simulink model "SICARO_STALL"  (R2022b)
settings: Solver=ode23t  StartTime=0.0  StopTime=84  MaxStep=1e-3  RelTol=1e-3  AbsTol=1e-3
values from neighbouring files (symbols this model uses):
  air_rho = 1.225    [sicaro_inherited_params(stall).mat]
  battery_capacity = 22.8    [sicaro_inherited_params(stall).mat]
  CDO = 10.25    [sicaro_inherited_params(stall).mat]
  drag_linear = 0.002    [sicaro_inherited_params(stall).mat]
  drag_quad = 0.005    [sicaro_inherited_params(stall).mat]
  filtD_motor = 100    [sicaro_inherited_params(stall).mat]
  filtSpd_motor = 0.001    [sicaro_inherited_params(stall).mat]
  flap_radius = 0.05312    [sicaro_inherited_params(stall).mat]
  flap_surface_area = 0.025    [sicaro_inherited_params(stall).mat]
  kd_motor = 0    [sicaro_inherited_params(stall).mat]
  ki_motor = 0.00045    [sicaro_inherited_params(stall).mat]
  klinear = 0.03    [sicaro_inherited_params(stall).mat]
  kquad = 0.025    [sicaro_inherited_params(stall).mat]
  limit_motor = 0.25    [sicaro_inherited_params(stall).mat]
  monoco_mass = 160    [sicaro_inherited_params(stall).mat]
  monoco_prop =     [sicaro_inherited_params(stall).mat]
  monoco_radius = 0.61    [sicaro_inherited_params(stall).mat]
  monoco_wing =     [sicaro_inherited_params(stall).mat]
  monoco_wing_area = 0.239    [sicaro_inherited_params(stall).mat]
  waypoints = [-2 -2 0.14 -2 -2 6 0 0 6 2 0 6 ... (15 elements, 3x5)]    [sicaro_inherited_params(stall).mat]
undefined symbols (not defined in the file or in its folder): X, Y, Z
libraries: sm_lib x96, nesl_utility x38, slpidlib x22, fl_lib x12, sdl_lib x3, simulink x2, simulink_extras x1, batteryecm_lib x1, ee_lib x1
(part 8 of 8)

== matlab function SICARO_STALL/Monowing/Monowing_Assem/Cyclic Command Distribution (Disk-Pitch Body-Roll) abt Yw ==
  data: azi input; quadrant input; flap_dihedral_pitch_cmd output; gain_disk_pitch input; Toggle input; Motor_Pulse output; desired_heading input
function [flap_dihedral_pitch_cmd,Motor_Pulse] = fcn(azi, quadrant, gain_disk_pitch, Toggle, desired_heading)

upper_bound = zeros(1,1);
lower_bound = zeros(1,1);
azimuth = azi;
heading = desired_heading;
pitch = zeros(1,1);
Motor_Pulse = zeros(1,1);
%% Quadrants anti clockwise fashion

if quadrant == 0 
    upper_bound = pi/2 + pi/4; 
    lower_bound = pi/2 - pi/4;
    if abs(azimuth) < upper_bound && abs(azimuth) > lower_bound
        tilt_xw = sin(azimuth); % tilt about yw heading in x direction 
        pitch = tilt_xw * gain_disk_pitch * -1; % only for cyclic y, -1 because craft is always pitching forward wrt to shifts in heading
        Motor_Pulse =  (pitch/abs(pitch)) * 1;
    else
        pitch = 0;
        Motor_Pulse = 0;
    end


elseif quadrant == 1
    upper_bound = (-pi/2) + heading + pi/4; 
    lower_bound = (-pi/2) + heading - pi/4;
    activate_cos = zeros(1,1);
    if lower_bound < -pi
        lower_bound = (lower_bound + pi) + pi;
        %lower_bound = -pi;
        activate_cos = 1;
    end
    if activate_cos == 0
        if (azimuth < upper_bound && azimuth > lower_bound) || (azimuth < pi + upper_bound && azimuth > pi + lower_bound) % otherside
            tilt_xw = sin(azimuth); % tilt about yw heading in x direction 
            pitch = tilt_xw * gain_disk_pitch * -1; % only for cyclic y, -1 because craft is always pitching forward wrt to shifts in heading
            Motor_Pulse =  (pitch/abs(pitch)) * 1;
        else
            pitch = 0;
            Motor_Pulse = 0;
        end
    else
        if azimuth < upper_bound || azimuth > lower_bound
            tilt_xw = cos(azimuth); % tilt about yw heading in x direction             
            pitch = tilt_xw * gain_disk_pitch * -1; % only for cyclic y, -1 because craft is always pitching forward wrt to shifts in heading
            Motor_Pulse =  (pitch/abs(pitch)) * 1;       
        elseif azimuth < upper_bound + pi && azimuth > lower_bound - pi % otherside
            tilt_xw = cos(azimuth); % tilt about yw heading in x direction 
            pitch = tilt_xw * gain_disk_pitch * -1; % only for cyclic y, -1 because craft is always pitching forward wrt to shifts in heading
            Motor_Pulse =  (pitch/abs(pitch)) * 1;
        else
            pitch = 0;
            Motor_Pulse = 0;
        end
    end

    
elseif quadrant == 1.5 
    upper_bound = pi + pi/4; 
    lower_bound = pi/4; 
    % no need for lower bound
    if abs(azimuth) > upper_bound || abs(azimuth) < lower_bound
        tilt_xw = cos(azimuth); % tilt about yw heading in x direction 
        pitch = tilt_xw * gain_disk_pitch * -1; % only for cyclic y, -1 because craft is always pitching forward wrt to shifts in heading 
        Motor_Pulse =  (pitch/abs(pitch)) * 1;
    else
        pitch = 0;
        Motor_Pulse = 0;
    end


elseif quadrant == 2
    upper_bound = pi/2 + heading + pi/4; 
    lower_bound = pi/2 + heading - pi/4;
    activate_cos = zeros(1,1); 

    if upper_bound > 0
        %lower_bound = (lower_bound + pi) + pi;
        %lower_bound = 0;
        activate_cos = 1;
    end

    if activate_cos == 0
        if (azimuth < upper_bound && azimuth > lower_bound) || (azimuth < pi + lower_bound && azimuth > pi + upper_bound) % otherside first
            tilt_xw = sin(azimuth); % tilt about yw heading in x direction 
            pitch = tilt_xw * gain_disk_pitch; % only for cyclic y
            Motor_Pulse =  (pitch/abs(pitch)) * 1;
        else
            pitch = 0;
            Motor_Pulse = 0;
        end
    else
        if azimuth > pi + lower_bound || azimuth < -(pi + upper_bound)
            tilt_xw = cos(azimuth); % tilt about yw heading in x direction 
            pitch = tilt_xw * gain_disk_pitch * -1; % only for cyclic y, -1 because craft is always pitching forward wrt to shifts in heading
            Motor_Pulse =  (pitch/abs(pitch)) * 1;
        elseif azimuth < upper_bound && azimuth > lower_bound
            tilt_xw = cos(azimuth); % tilt about yw heading in x direction 
            pitch = tilt_xw * gain_disk_pitch * -1; % only for cyclic y, -1 because craft is always pitching forward wrt to shifts in heading
            Motor_Pulse =  (pitch/abs(pitch)) * 1;
        else
            pitch = 0;
            Motor_Pulse = 0;
        end
    end


elseif quadrant == 2.5
    upper_bound = pi/2 + pi/4; 
    lower_bound = pi/2 - pi/4;
    if abs(azimuth) < upper_bound && abs(azimuth) > lower_bound
        tilt_xw = sin(azimuth); % tilt about yw heading in x direction 
        pitch = tilt_xw * gain_disk_pitch; % only for cyclic y
        Motor_Pulse =  (pitch/abs(pitch)) * 1;
    else
        pitch = 0;
        Motor_Pulse = 0;
    end


elseif quadrant == 3
    upper_bound = (-pi/2) + heading + pi/4; 
    lower_bound = (-pi/2) + heading - pi/4;
    activate_cos = zeros(1,1);  
    if lower_bound < 0
        %lower_bound = (lower_bound + pi) + pi;
        activate_cos = 1;
    end

    if activate_cos == 0
        if (azimuth < upper_bound && azimuth > lower_bound) || (azimuth > -pi + lower_bound && azimuth < -pi + upper_bound) % otherside first
            tilt_xw = sin(azimuth); % tilt about yw heading in x direction 
            pitch = tilt_xw * gain_disk_pitch * -1; % only for cyclic y
            Motor_Pulse =  (pitch/abs(pitch)) * 1;
        else
            pitch = 0;
            Motor_Pulse = 0;
        end  
    else
        if azimuth < upper_bound && azimuth > lower_bound
            tilt_xw = cos(azimuth); % tilt about yw heading in x direction 
            pitch = tilt_xw * gain_disk_pitch * -1; % only for cyclic y
            Motor_Pulse =  (pitch/abs(pitch)) * 1;
        elseif azimuth > pi - lower_bound || azimuth < -pi + upper_bound % otherside first
            tilt_xw = cos(azimuth); % tilt about yw heading in x direction 
            pitch = tilt_xw * gain_disk_pitch * -1; % only for cyclic y
            Motor_Pulse =  (pitch/abs(pitch)) * 1;
        else
            pitch = 0;
            Motor_Pulse = 0;
        end 
    end


elseif quadrant == 3.5
    upper_bound = pi + pi/4; 
    lower_bound = pi/4; 
    % no need for lower bound
    if abs(azimuth) > upper_bound || abs(azimuth) < lower_bound
        tilt_xw = cos(azimuth); % tilt about yw heading in x direction 
        pitch = tilt_xw * gain_disk_pitch * -1;
        Motor_Pulse =  (pitch/abs(pitch)) * 1;
    else
        pitch = 0;
        Motor_Pulse = 0;
    end


elseif quadrant == 4
    upper_bound = pi/2 + heading + pi/4; 
    lower_bound = pi/2 + heading - pi/4;
    activate_cos = zeros(1,1); 

    if upper_bound > 0
        %lower_bound = (lower_bound + pi) + pi;
        %lower_bound = 0;
        activate_cos = 1;
    end

    if activate_cos == 0
        if (azimuth < upper_bound && azimuth > lower_bound) || (azimuth > -pi + lower_bound && azimuth < -pi + upper_bound) % otherside first
            tilt_xw = sin(azimuth); % tilt about yw heading in x direction 
            pitch = tilt_xw * gain_disk_pitch * -1; % only for cyclic y, -1 because craft is always pitching forward wrt to shifts in heading
            Motor_Pulse =  (pitch/abs(pitch)) * 1;
        else
            pitch = 0;
            Motor_Pulse = 0;
        end
    else
         if azimuth > lower_bound || azimuth < -pi + upper_bound - pi
            tilt_xw = cos(azimuth); % tilt about yw heading in x direction 
            pitch = tilt_xw * gain_disk_pitch * -1; % only for cyclic y
            Motor_Pulse =  (pitch/abs(pitch)) * 1;
         elseif azimuth < upper_bound - pi && azimuth > -pi + lower_bound
            tilt_xw = cos(azimuth); % tilt about yw heading in x direction 
            pitch = tilt_xw * gain_disk_pitch * -1; % only for cyclic y
            Motor_Pulse =  (pitch/abs(pitch)) * 1;
         else
            pitch = 0;
            Motor_Pulse = 0;
         end
    end

else
    Motor_Pulse =  0;
    pitch = 0;
end


if Toggle == 1 % Front Motor    
    if abs(pitch) > 0.4
        pitch = (pitch/abs(pitch)) * 0.4;
    end
elseif Toggle == 0
    Motor_Pulse =  0;
    pitch = 0;
end

flap_dihedral_pitch_cmd = pitch;

% elseif Toggle == 2 % Back Motor
% 
%     azimuth = azi;
%     if (abs(azimuth) > pi/4) && (abs(azimuth) < 3*pi/4)
%         tilt_xw = sin(azimuth + heading); % tilt around xw heading in y direction 
%         pitch = zeros(1,1);
%         pitch = tilt_xw * gain_disk_pitch; % only for cyclic y
%         Motor_Pulse =  (pitch/abs(pitch)) * 1;
% 
%         if abs(pitch) > 0.75
%             pitch = (pitch/abs(pitch)) * 0.75;
%         end
% 
%         flap_dihedral_pitch_cmd = pitch;
% 
%     else
%         
%         Motor_Pulse =  0;
%         flap_dihedral_pitch_cmd = 0.0;
% 
%     end
% 
% else
%     
%     Motor_Pulse =  0;
%     flap_dihedral_pitch_cmd = 0.0;












% if Toggle == 1 % Front Motor
% 
%     azimuth = azi;
%     %heading = deg2rad(heading);
%     if (abs(azimuth - heading) < pi/4) || (abs(azimuth - heading) > 3*pi/4)
%         tilt_xw = sin(azimuth - heading); % tilt about yw heading in x direction 
%         pitch = zeros(1,1);
%         pitch = tilt_xw * gain_disk_pitch; % only for cyclic y
%         Motor_Pulse =  (pitch/abs(pitch)) * 1;
% 
%         if abs(pitch) > 0.60
%             pitch = (pitch/abs(pitch)) * 0.60;
%         end
% 
%         flap_dihedral_pitch_cmd = pitch;
% 
%     else
%         
%         Motor_Pulse =  0;
%         flap_dihedral_pitch_cmd = 0.0;
% 
%     end
% 
% elseif Toggle == 2 % Back Motor
% 
%     azimuth = azi;
%     if (abs(azimuth) > pi/4) && (abs(azimuth) < 3*pi/4)
%         tilt_xw = sin(azimuth + heading); % tilt around xw heading in y direction 
%         pitch = zeros(1,1);
%         pitch = tilt_xw * gain_disk_pitch; % only for cyclic y
%         Motor_Pulse =  (pitch/abs(pitch)) * 1;
% 
%         if abs(pitch) > 0.75
%             pitch = (pitch/abs(pitch)) * 0.75;
%         end
% 
%         flap_dihedral_pitch_cmd = pitch;
% 
%     else
%         
%         Motor_Pulse =  0;
%         flap_dihedral_pitch_cmd = 0.0;
% 
%     end
% 
% else
%     
%     Motor_Pulse =  0;
%     flap_dihedral_pitch_cmd = 0.0;
% 
% end





% kp = 1.3;
% desired_roll = 10;
% if (Annular_roll/abs(Annular_roll)) > 0.0
%     error_gain = kp*(Annular_roll - desired_roll);
% 
% elseif (Annular_roll/abs(Annular_roll)) < 0.0
%     error_gain = kp*(Annular_roll - (-1*desired_roll));
% 
% else
%     error_gain = 0.0;
% 
% end

% roll = gain * desired_flap * 2; % only for cyclic (original) 
% roll = desired_flap; % collective
% flap_cmd = roll - error_gain;

== matlab function SICARO_STALL/Monowing/Quat2Eul Function ==
  data: u input; Euler_Angles_Collectively output size=[1 4] [-1000..1000]; bod_pitch_deg_abt_Xb output size=[1,1]; bod_roll_deg_abt_Yb output; body_yaw_rad_z output; Pos output size=[1 5]; Time input; pos_x input; pos_y input; pos_z input; rps input
function [Euler_Angles_Collectively, bod_pitch_deg_abt_Xb, bod_roll_deg_abt_Yb, body_yaw_rad_z, Pos] = fcn(u, Time, pos_x, pos_y, pos_z, rps)
coder.extrinsic('quat2eul');
anx = zeros(1,3);
dax = zeros(1,3);
body_pitch_deg = zeros(1,1);
body_roll_deg = zeros(1,1);
yaw_rad = zeros(1,1);
default_heading = zeros(1,1); % zero heading is at body yb facing world yw 
quat = flip(transpose(u));
% disp (quat);

eul = quat2eul(quat); % ZYX 
% Z = zeros(1,1);

% Body frame dynamics
Z = eul(1,1);
Y = eul(1,2);
X = eul(1,3);
body_pitch_deg = rad2deg(X);
body_roll_deg = rad2deg(Y);
% yaw_deg = rad2deg(Z);
yaw_rad = Z;

anx = rad2deg([X Y Z]);
Pos = [Time pos_x pos_y pos_z rps];
% disp (size(deg));
% disp (size(Z));
Euler_Angles_Collectively = [Time, anx];

% World frame dynamics
% annular_pitch_deg_abt_yw = -1*body_pitch_deg; % anti clockwise is negative but i negate it so its easier to read; annular y axis in world frame
% annular_roll_deg_abt_xw = 1*body_roll_deg; % clockwise is positive; annular x axis in world frame

% Body frame dynamics in euler
bod_pitch_deg_abt_Xb = -1*body_pitch_deg;
bod_roll_deg_abt_Yb = 1*body_roll_deg;
body_yaw_rad_z = yaw_rad;

% Disk frame dynamics in euler (ZYX)
dax = deg2rad([0 bod_roll_deg_abt_Yb 0]);

== matlab function SICARO_STALL/Cyclic Roll Control/Velocity Feedback ==
  data: vel_mag_feedback output; Y_fb input; X_fb input
function vel_mag_feedback  = fcn(Y_fb,X_fb)

velfb = zeros(1,1);
velfb = sqrt(Y_fb^2 + X_fb^2);
vel_mag_feedback = velfb;

== matlab function SICARO_STALL/Cyclic Roll Control/PD Control (Vel)/Gain Switching ==
  data: aggro input; y output; annular_roll input; gentle input; Toggle input
function y = fcn(aggro, annular_roll, gentle,Toggle)

if Toggle > 0
    if abs(annular_roll) > 5
        y = aggro;
    else
        y = gentle;
    end
else
    y = 0;
end

% y = gentle;

== matlab function SICARO_STALL/Cyclic Roll Control/Acc Feedback Calculation ==
  data: z_d output; xy_feedback input; z_feedback input; a_xy_ref input; pitch input
function z_d   = fcn(xy_feedback,z_feedback,a_xy_ref,pitch)

xy_des = zeros(1,1);
z_des = zeros(1,1);
g = 9.81;
mea_euler = [0,0,abs(deg2rad(pitch))]; % default seq is ZYX
ez = [0,0,1];
aux = Sim_AuxiliaryFunctions;
circle = aux.circle_setpoints(1,-2,-2,1);
ref_pos = circle(1,:);
ref_vel = circle(2,:);
ref_acc = circle(3,:);
ref_jer = circle(4,:);
ref_sna = circle(5,:);
ref_dir = circle(6,:);
time_per_setpt = circle(7,1);

% A_Des
xy_des = xy_feedback + a_xy_ref;
z_des = z_feedback - g;
a_des = [xy_des,0,z_des];

% ZD
z_d = a_des/norm(a_des);

% Disk_Vector 
qz = eul2quat(mea_euler); % default seq is ZYX
d_v = quatrotate(qz,ez);
angle = acos(dot(d_v,z_d)/(norm(disk_vector)*(norm(zd))));

% Body_rates
n = cross(d_v,zd) / norm(cross(d_v,zd));
B = quatrotate((quatinv(qz)),n); 
error_quat = [cos(angle/2),B*sin(angle/2)];
prp = zeros(1,2);

if error_quat(:,1) < 0
    body_rates = -2 * (1/time_per_setpt) * prp * error_quat(:,2:3); % default seq is q = [w x y z]
else
    body_rates = 2 * (1/time_per_setpt) * prp * error_quat(:,2:3); % default seq is q = [w x y z]
end

%% To be continued...
% cmd_bodyrate = ppq * (body_rates(:,2) - mea_pitch_rate) * 1/time_per_setpt; % gain for cyclic, multiply this to azimuth sin or cos from quadrant, the other value is the desired heading  
% 
% % Collective thrust
% cmd_z = dot(transpose(zd),transpose(a_des)); %% command sent to motor, need to include filter to make sure negative cmds dun go thru

== matlab function SICARO_STALL/Monowing/Monowing_Assem/Old SICARO Controller For Translation/Collective & Cyclic Command Distribution (Transition) ==
  data: stalling_flap input; flap_transition_cmd output; Time input; Toggle input
function flap_transition_cmd = fcn(stalling_flap,Time, Toggle)
if Toggle == 1
    
    roll = zeros(1,1);
    roll = stalling_flap; % collective
    
    if Time > 8.0
        flap_transition_cmd = 0.0;
    else 
        flap_transition_cmd = roll;
    end

else

    flap_transition_cmd = 0.0;

end

== matlab function SICARO_STALL/Monowing/Drag moment/Drag Moment (X & Y) ==
  data: y input; drag_moment_abt_y output; drag_linear parameter; drag_quad parameter; x input; drag_moment_abt_x output; azimuth input
function [drag_moment_abt_y,drag_moment_abt_x] = fcn(y, drag_linear, drag_quad, x, azimuth)
drag_moment_y  = zeros(1,1);
drag_moment_x  = zeros(1,1);
gain = cos(azimuth);
drag_moment_y = (drag_linear * y) + (drag_quad * y^2); 
drag_moment_x = (drag_linear * x) + (drag_quad * x^2); 

drag_moment_abt_y = -1 * drag_moment_y;
drag_moment_abt_x = -1 * drag_moment_x;

== matlab function SICARO_STALL/Monowing/Horizontal Forces/Horizontal Motion Y ==
  data: roll_in_deg input; force output; Lift input; flap_angle_data input; flap_angle_recording output; vx input; vy input; vz input; klinear parameter; kquad parameter; y_force_percentage input; azimuth input; flap_angle input; quadrant input; gain input; active_state output
function [force, flap_angle_recording,active_state] = fcn(roll_in_deg, Lift, flap_angle_data, vx, vy, vz, klinear, kquad, y_force_percentage, azimuth, flap_angle, quadrant,gain)
fy = zeros(1,1);
y = zeros(1,1);
v_l1 = zeros(1,1);
v_l2 = zeros(1,1);
roll_angle = abs(roll_in_deg);
%disp(Lift);
dihedral_offset = 2.0;
v_l1 = abs(vx) + abs(vy) + abs(vz);
v_l2 = sqrt(vx^2 + vy^2 + vz^2);

negative_y = 0;
positive_y = 1;
neutral_y = 2;
active_state = 0;
% if abs(azimuth) < pi/2 && flap_angle > 0 
%     current_state = negative_y; % positive y with z axis facing in
%     active_state = 1;
%     
% elseif abs(azimuth) > pi/2 && flap_angle < 0
%     current_state = negative_y; % positive y with z axis facing in
%     active_state = 2;
% 
% elseif abs(azimuth) > pi/2 && flap_angle > 0
%     current_state = positive_y; % negative y with z axis facing in
%     active_state = 3;
% 
% elseif abs(azimuth) < pi/2 && flap_angle < 0
%     current_state = positive_y; % negative y with z axis facing in
%     active_state = 4;
% 
% else
%     current_state = neutral_y;
%     active_state = 0;
% end

%% to be continued
if quadrant == 1.5 || quadrant == 2 || quadrant == 3.5 || quadrant == 4
    if abs(gain) > 0
        current_state = positive_y;
    else
        current_state = neutral_y;
    end
%     if gain > 0
%        current_state = positive_y; % positive means negative in my eqn 
%        active_state = 0;
%     elseif gain < 0 
%        current_state = negative_y; % vice versa as of the above
%        active_state = 1;
%     else
%        current_state = neutral_y;
%        active_state = 2;
%     end

elseif quadrant == 0 || quadrant == 2.5
    current_state = neutral_y;

% elseif quadrant == 3 || quadrant == 3.5
%     if abs(gain) > 0
%         current_state = negative_y;
%     else
%         current_state = neutral_y;
%     end
        %     if gain > 0
%        current_state = negative_y; % positive means negative in my eqn 
%     elseif gain < 0 
%        current_state = positive_y; 
%     else
%        current_state = neutral_y;
%     end

elseif quadrant == 3 || quadrant == 1 
    if abs(gain) > 0
        current_state = negative_y;
    else
        current_state = neutral_y;
    end

else
    current_state = neutral_y; 

end



% disp (current_state);
% disp (azimuth);
% disp (flap_angle);

% current_state = negative_y;

switch(current_state)
    % positive y with z axis facing in  
    case negative_y %%% this is a function of the roll angle and therefore if the roll angle amplifies, it wud go haywire
        if roll_in_deg > 0 && roll_in_deg > dihedral_offset 
%             if roll_in_deg > 0
            fy = Lift*sind(roll_in_deg-dihedral_offset);
            y = (-0.3*fy) + (kquad*v_l1*abs(vy) + klinear*abs(vy));
            y = gain / abs(gain) * y * y_force_percentage;
            active_state = -1;
        elseif roll_in_deg < 0
            fy = Lift*sind(roll_angle);
            y = (-0.3*fy) + (kquad*v_l1*abs(vy) + klinear*abs(vy));
            %y = y  (kquad*v_l1*abs(vy) + klinear*abs(vy));
            y = gain / abs(gain) * y * y_force_percentage;
            active_state = -2;
        else
            y = 0.0;
        end
    % negative y with z axis facing in
    case positive_y
        if roll_in_deg > 0 && roll_in_deg > dihedral_offset 
        %     if roll_in_deg > 0
            fy = Lift*sind(roll_in_deg-dihedral_offset);
            y = fy - (kquad*v_l1*abs(vy) + klinear*abs(vy));
            y = gain / abs(gain) * y * y_force_percentage;
            active_state = 1;
        elseif roll_in_deg < 0
            fy = Lift*sind(roll_angle);
            y = fy - (kquad*v_l1*abs(vy) + klinear*abs(vy));
            %y = y  (kquad*v_l1*abs(vy) + klinear*abs(vy));
            y = gain / abs(gain)* y * y_force_percentage;
            active_state = 2;
        else
            y = 0.0;
        end

    case neutral_y 
            y = 0.0;

end

force = y;
% Acceleration_in_y_axis = y/monoco_mass;
flap_angle_recording = flap_angle_data;

== matlab function SICARO_STALL/Monowing/Collective Control/Collective (Dihedral) ==
  data: Torque_negative input; output output; Toggle input
function output  = fcn(Torque_negative,Toggle)

if Toggle == 1 
    output = Torque_negative;
else
    output = 0;
end
